simulink model "motor_pos_str"  (R2018a)
settings: Solver=FixedStepAuto  StartTime=0.0  StopTime=20  FixedStep=0.005  RelTol=1e-3
settings Model: Creator=DELL  LastModifiedBy=DELL

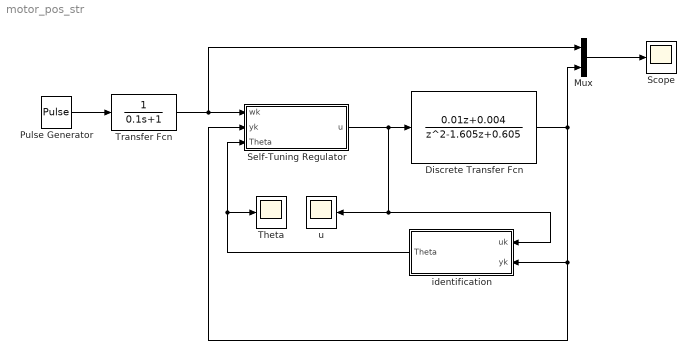
== system motor_pos_str ==
  Discrete Transfer Fcn : DiscreteTransferFcn  Numerator=[0.01 0.004]  Denominator=[1 -1.605 0.605]  SampleTime=0.005
  Mux : Mux  Inputs=2
  Pulse Generator : DiscretePulseGenerator  PulseType=Time based  Period=4  PulseWidth=50
  Scope : Scope
  Self-Tuning Regulator : Subsystem
  Theta : Scope
  Transfer Fcn : TransferFcn  Denominator=[0.1 1]
  identification : Subsystem
  u : Scope
  wires:
  Pulse Generator/1 -> Transfer Fcn/1
  Mux/1 -> Scope/1
  Self-Tuning Regulator/1(u) -> u/1, identification/1(uk), Discrete Transfer Fcn/1
  Transfer Fcn/1 -> Mux/1, Self-Tuning Regulator/1(wk)
  Discrete Transfer Fcn/1 -> Mux/2, identification/2(yk), Self-Tuning Regulator/2(yk)
  identification/1(Theta) -> Theta/1, Self-Tuning Regulator/3(Theta)

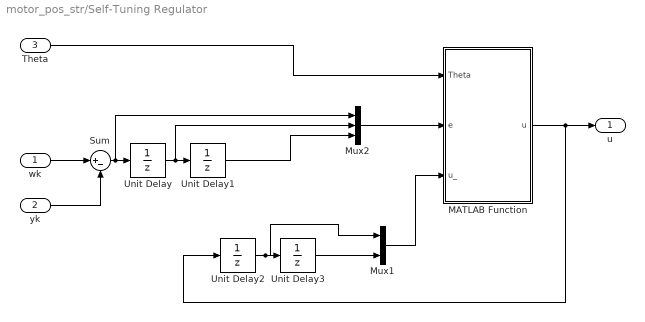
== system motor_pos_str/Self-Tuning Regulator ==
  wk : Inport
  yk : Inport  Port=2
  Theta : Inport  Port=3
  MATLAB Function : MATLAB Function  TreatAsAtomicUnit=on
  Mux1 : Mux  Inputs=2
  Mux2 : Mux  Inputs=3
  Sum : Sum  Inputs=|+-
  Unit Delay{,1..3} (4 alike) : UnitDelay  SampleTime=-1
  u : Outport
  wires:
  wk/1 -> Sum/1
  yk/1 -> Sum/2
  Sum/1 -> Mux2/1, Unit Delay/1
  Unit Delay/1 -> Mux2/2, Unit Delay1/1
  Unit Delay2/1 -> Mux1/1, Unit Delay3/1
  Unit Delay3/1 -> Mux1/2
  Theta/1 -> MATLAB Function/1(Theta)
  Mux1/1 -> MATLAB Function/3(u_)
  Unit Delay1/1 -> Mux2/3
  Mux2/1 -> MATLAB Function/2(e)
  MATLAB Function/1(u) -> u/1, Unit Delay2/1

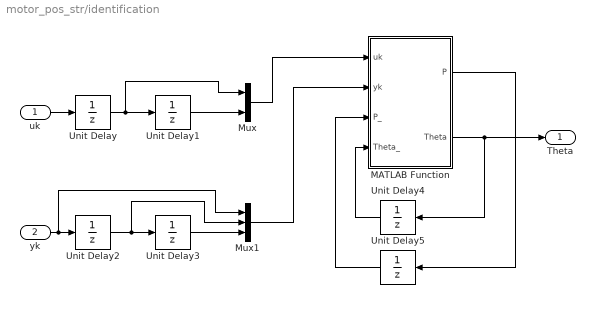
== system motor_pos_str/identification ==
  uk : Inport
  yk : Inport  Port=2
  MATLAB Function : MATLAB Function  TreatAsAtomicUnit=on
  Mux : Mux  Inputs=2
  Mux1 : Mux  Inputs=3
  Unit Delay{,1..5} (6 alike) : UnitDelay  SampleTime=-1
  Theta : Outport
  wires:
  yk/1 -> Mux1/1, Unit Delay2/1
  uk/1 -> Unit Delay/1
  Unit Delay/1 -> Mux/1, Unit Delay1/1
  Unit Delay1/1 -> Mux/2
  Unit Delay3/1 -> Mux1/3
  Unit Delay2/1 -> Mux1/2, Unit Delay3/1
  MATLAB Function/2(Theta) -> Unit Delay4/1, Theta/1
  MATLAB Function/1(P) -> Unit Delay5/1
  Unit Delay4/1 -> MATLAB Function/4(Theta_)
  Unit Delay5/1 -> MATLAB Function/3(P_)
  Mux1/1 -> MATLAB Function/2(yk)
  Mux/1 -> MATLAB Function/1(uk)

== matlab function motor_pos_str/Self-Tuning Regulator/MATLAB Function ==
  data: Theta input; u output; e input; u_ input
% Ham tinh thong so bo dieu khien theo pp dat cuc lien tuc
function u = STR_pp1(Theta,e,u_)

T0 = 0.005;
xi = 0.9;
wn = 50;

% Gan lai thong so de thuan tien viec tinh toan
a1 = Theta(1);
a2 = Theta(2);
b1 = Theta(3);
b2 = Theta(4);

% Tinh thong so bo dieu khien
if(xi<1)
d1 = -2*exp(-xi*wn*T0)*cos(wn*T0*sqrt(1-xi^2)); % xi<1
else
d1 = -2*exp(-xi*wn*T0)*cosh(wn*T0*sqrt(xi^2-1)); % xi>1
end
d2 = exp(-2*xi*wn*T0);
r1 = (b1+b2)*(a1*b1*b2-a2*b1^2-b2^2);
s1 = a2*((b1+b2)*(a1*b2-a2*b1)+b2*(b1*d2-b2*d1-b2));
q2 = s1/r1;
gama = q2*b2/a2;
q1 = a2/b2-q2*(b1/b2-a1/a2+1);
q0 = 1/b1*(d1+1-a1-gama);

% Luat dieu khien
u = q0*e(1) + q1*e(2) + q2*e(3) + (1-gama)*u_(1) + gama*u_(2);

== matlab function motor_pos_str/identification/MATLAB Function ==
  data: uk input; P output; yk input; P_ input; Theta_ input; Theta output
function [P,Theta] = Uocluong(uk,yk,P_,Theta_)
lamda = 0.96;
PHI = [-yk(2); -yk(3); uk(1); uk(2)];
e = yk(1) - PHI'*Theta_;
L = P_*PHI / (lamda + PHI'*P_*PHI);
P = 1/lamda*(P_ - P_*PHI*PHI'*P_ /(lamda + PHI'*P_*PHI));
Theta = Theta_ + L*e;
